simulink model "Question_3_simulink"  (R2021a)
settings: Solver=VariableStepAuto  StartTime=0.0  StopTime=10.0  RelTol=1e-3
InitFcn:
  | sysvar
values from neighbouring files (symbols this model uses):
  d = 8    [sysvar.m]
  f = 6    [sysvar.m]
  f1 = 1    [sysvar.m]
  f2 = -1    [sysvar.m]
  f3 = 10    [sysvar.m]
  m1 = 1    [sysvar.m]
  m2 = 1.5    [sysvar.m]
settings Model: Creator=my computer  LastModifiedBy=my computer

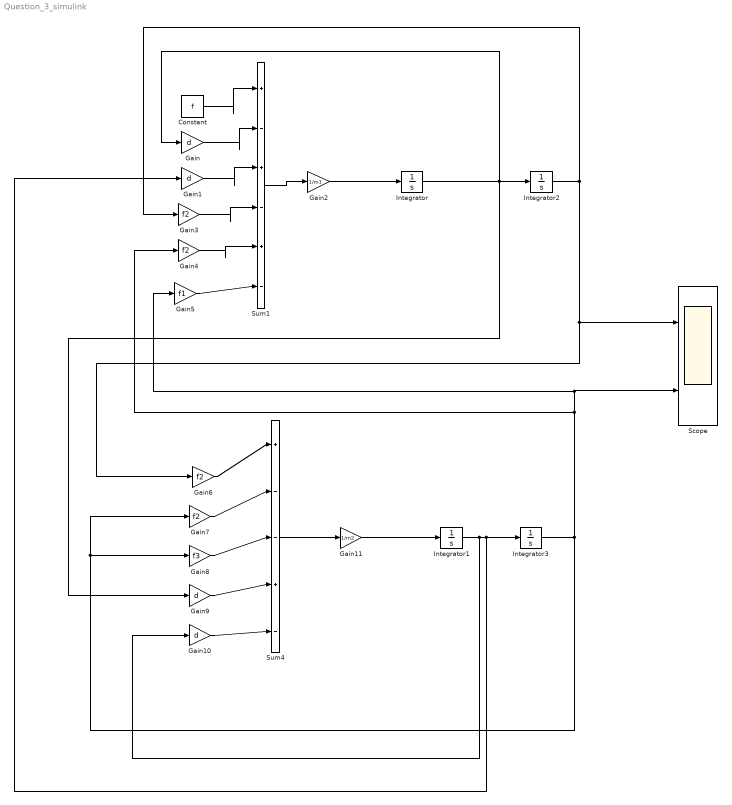
== system Question_3_simulink ==
  Constant : Constant  Value=f
  Gain{,1,9..10} (4 alike) : Gain  Gain=d
  Gain11 : Gain  Gain=1/m2
  Gain2 : Gain  Gain=1/m1
  Gain{3..4,6..7} (4 alike) : Gain  Gain=f2
  Gain5 : Gain  Gain=f1
  Gain8 : Gain  Gain=f3
  Integrator{,1..3} (4 alike) : Integrator
  Scope : Scope  NumInputPorts=2
  Sum1 : Sum  Inputs=|+-+-+-
  Sum4 : Sum  Inputs=|+--+-
  wires:
  Constant/1 -> Sum1/1
  Gain/1 -> Sum1/2
  Gain1/1 -> Sum1/3
  Sum1/1 -> Gain2/1
  Gain2/1 -> Integrator/1
  Integrator2/1 -> Gain6/1, Scope/1, Gain3/1
  Integrator/1 -> Gain9/1, Gain/1, Integrator2/1
  Gain3/1 -> Sum1/4
  Gain4/1 -> Sum1/5
  Gain5/1 -> Sum1/6
  Gain6/1 -> Sum4/1
  Gain7/1 -> Sum4/2
  Gain8/1 -> Sum4/3
  Gain9/1 -> Sum4/4
  Gain10/1 -> Sum4/5
  Sum4/1 -> Gain11/1
  Gain11/1 -> Integrator1/1
  Integrator1/1 -> Gain10/1, Gain1/1, Integrator3/1
  Integrator3/1 -> Gain5/1, Scope/2, Gain4/1, Gain7/1, Gain8/1
